simulink model "code_hinfinity"  (R2023b)
settings: Solver=VariableStepAuto  StartTime=0.0  StopTime=5  RelTol=1e-3
libraries: cstblocks x2
settings Model: Creator=DELL  LastModifiedBy=DELL
settings DebuggingCC: UnconnectedInputMsg=warning  UnconnectedOutputMsg=warning  UnconnectedLineMsg=warning
settings ModelReferenceCC: EnableRefExpFcnMdlSchedulingChecks=on
settings RTWCC: DLArmComputeVersion=19.05

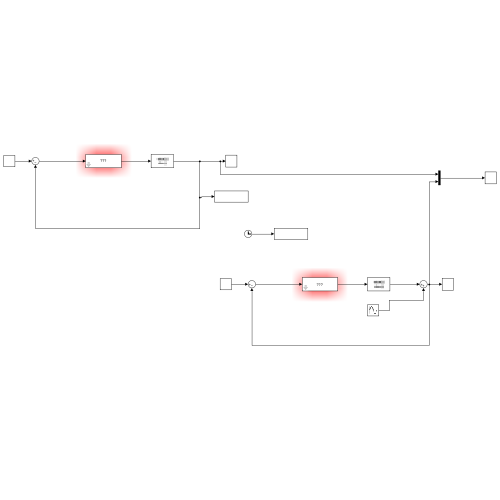
[thumbnail: Simulink's stored preview of the top-level diagram]
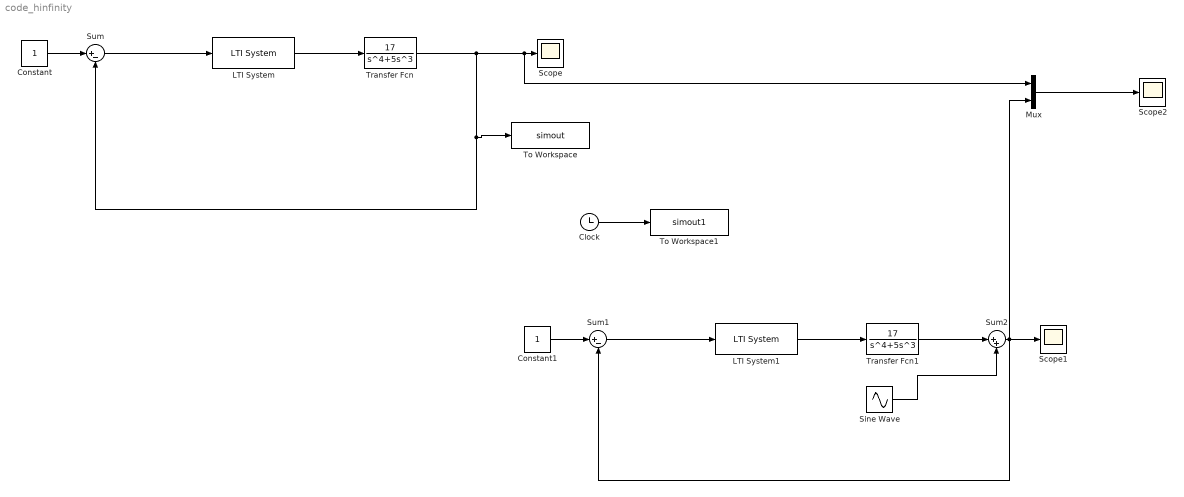
== system code_hinfinity ==
  Clock : Clock
  Constant : Constant
  Constant1 : Constant
  LTI System : cstblocks/LTI System  sys=K_tf  IC=[]  PadeOrder=0
  LTI System1 : cstblocks/LTI System  sys=K_tf  IC=[]  PadeOrder=0
  Mux : Mux  Inputs=2
  Scope : Scope
  Scope1 : Scope
  Scope2 : Scope
  Sine Wave : Sin  Amplitude=0.05  Frequency=0.5  SampleTime=0
  Sum : Sum  Inputs=|+-
  Sum1 : Sum  Inputs=|+-
  Sum2 : Sum  Inputs=|++
  To Workspace : ToWorkspace  VariableName=simout  SaveFormat=Timeseries
  To Workspace1 : ToWorkspace  VariableName=simout1  SaveFormat=Timeseries
  Transfer Fcn : TransferFcn  Numerator=17  Denominator=[1 5 0 0 0]
  Transfer Fcn1 : TransferFcn  Numerator=17  Denominator=[1 5 0 0 0]
  wires:
  LTI System/1 -> Transfer Fcn/1
  Constant/1 -> Sum/1
  Sum/1 -> LTI System/1
  Transfer Fcn/1 -> To Workspace/1, Sum/2, Mux/1, Scope/1
  Sum1/1 -> LTI System1/1
  Constant1/1 -> Sum1/1
  LTI System1/1 -> Transfer Fcn1/1
  Transfer Fcn1/1 -> Sum2/1
  Sum2/1 -> Sum1/2, Mux/2, Scope1/1
  Sine Wave/1 -> Sum2/2
  Mux/1 -> Scope2/1
  Clock/1 -> To Workspace1/1
